simulink model "ECE552ProjectSim"  (R2018b)
settings: Solver=ode45  StartTime=0.0  StopTime=43200  RelTol=1e-3  EnableMultiTasking=on
undefined symbols (not defined in the file or in its folder): Acid, Lead, sigbuilder_block
libraries: powerlib x3, electricdrivelib x1, powerlib_meascontrol x1
settings Model: Creator=kegarcia  LastModifiedBy=cluck
settings SolverCC: ZeroCrossControl=DisableAll
settings DataIOCC: LimitDataPoints=on  SaveFormat=Array
settings OptimizationCC: LifeSpan=inf  SimCompilerOptimization=on
settings DebuggingCC: AlgebraicLoopMsg=none  MaxConsecutiveZCsMsg=none  SFUnexpectedBacktrackingDiag=warning  SFNoUnconditionalDefaultTransitionDiag=warning  SFExecutionAtInitializationDiag=none
settings HardwareCC: ProdBitPerPointer=32  ProdBitPerSizeT=32  ProdBitPerPtrDiffT=32  ProdLargestAtomicFloat=None  ProdIntDivRoundTo=Undefined  ProdEndianess=Unspecified  ProdWordSize=32  ProdHWDeviceType=32-bit Generic
settings ModelReferenceCC: PropagateSignalLabelsOutOfModel=off
settings SFSimCC: SimUseLocalCustomCode=off
settings RTWCC: RTWUseLocalCustomCode=off
settings CodeAppCC: StateflowObjectComments=on
settings GRTTargetCC: TargetLangStandard=C89/C90 (ANSI)  GeneratePreprocessorConditionals=Disable all
settings ConfigComp: CovMetricSettings=dw  CovHtmlReporting=on  CovSaveCumulativeToWorkspaceVar=on  CovSaveSingleToWorkspaceVar=on  CovExternalEMLEnable=off
settings SimscapeCC: SimscapeNormalizeSystem=off

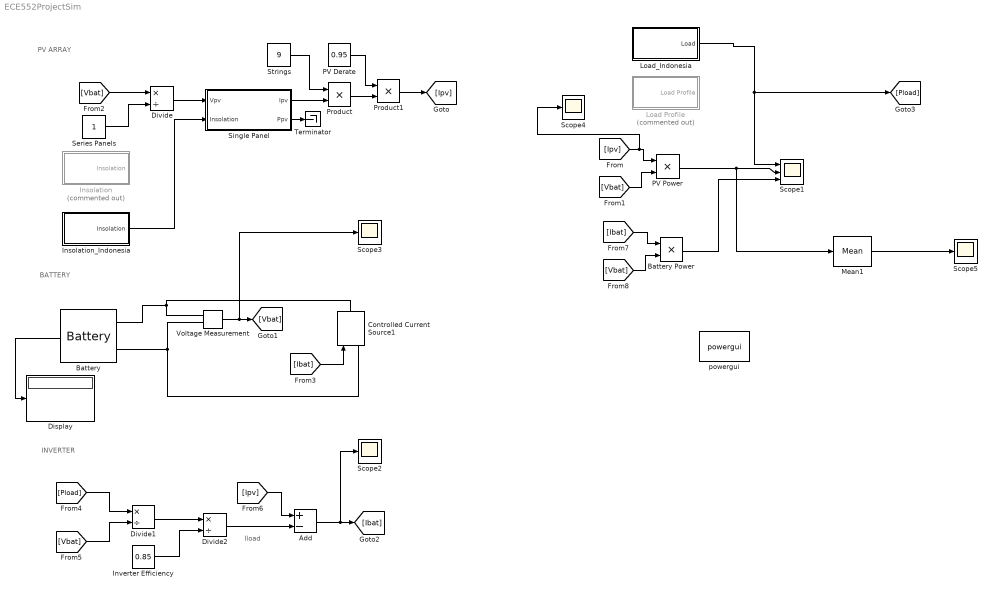
== system ECE552ProjectSim ==
  note: Iload
  note: INVERTER
  note: PV ARRAY
  note: BATTERY
  " Series Panels " : Constant
  " Strings" : Constant  Value=9
  Add : Sum  Inputs=+-
  Battery : electricdrivelib/Extra Sources/Battery  BatType=Lead-Acid  ShowTempParam=off  ThermalPreset=no  ShowAgeParam=off  NomV=24  NomQ=1200  SOC=95  Batt_Tr=30  PresetModel=off  MaxQ=1500  MinV=18  FullV=28  Dis_rate=5  R=0.0018462  Normal_OP=1200  expZone="[27        1500]"  current=[6.5 13 32.5]  Units=Time  Tci=20  NomT=20  T2=-30  MaxQ2=4.8  FullV2=7.1  Normal_OP2=5.655  expZone2="[6.58           1]"  Rca=0.6  ti=2000  Dp=0  Neq0=0  Tsim=1e6  Ta1=25  Qeol=5.4*0.9  Reol=0.013333*1.2  Char_age=[2.3478, 3]  Dis_age=[2.3478, 10]  N1=1500  N2=10500  N3=1000  N4=1400  Ta2=45  N5=950
      settings: SourceProductName=Simscape Electrical
  Battery Power : Product
  Controlled Current Source1 : powerlib/Electrical Sources/Controlled Current Source  Initialize=on  Source_Type=AC  Amplitude=0  Phase=0  Frequency=0  Measurements=None
      settings: SourceProductName=Simscape Electrical
  Display : Display
  Divide : Product  Inputs=*/
  Divide1 : Product  Inputs=*/
  Divide2 : Product  Inputs=*/
  Insolation : Subsystem  Tag=STV Subsys  Commented=on  LoadFcn=sigbuilder_block('load');  StartFcn=sigbuilder_block('start');  StopFcn=sigbuilder_block('stop');  ClipboardFcn=sigbuilder_block('clipboard');  mask(Sigbuilder block){tuvar=[0:10]}
      mask help: Simulink:masks:SigbuilderBlock_MD
      mask init:
      | if ~strcmp(get_param(bdroot(gcbh),'SimulationStatus'),'stopped') tuvar = sigbuilder_block('maskInit'); end
      settings: CopyFcn=sigbuilder_block('copy');  DeleteFcn=sigbuilder_block('delete');  ModelCloseFcn=sigbuilder_block('modelClose');  PreSaveFcn=sigbuilder_block('preSave');  PauseFcn=sigbuilder_block('pause')  ContinueFcn=sigbuilder_block('continue')  NameChangeFcn=sigbuilder_block('namechange');  OpenFcn=sigbuilder_block('open',[5.5 42.5 949 437.5 ]);  CloseFcn=sigbuilder_block('close');
      mask Display: plot(0, 0, 100, 100,[2, 2, 32, 32, 2], [68, 8, 8, 68, 68],[32, 2], [38, 38], [32, 19, 2],[53, 60, 44], [32, 17, 17, 2],[16, 16, 31, 31]);txt = getActiveGroup(gcbh);text(2, 100, txt,'verticalAlignment', 'top');
  Insolation_Indonesia : Subsystem  Tag=STV Subsys  LoadFcn=sigbuilder_block('load');  StartFcn=sigbuilder_block('start');  StopFcn=sigbuilder_block('stop');  ClipboardFcn=sigbuilder_block('clipboard');  mask(Sigbuilder block){tuvar=[0:10]}
      mask help: Simulink:masks:SigbuilderBlock_MD
      mask init:
      | if ~strcmp(get_param(bdroot(gcbh),'SimulationStatus'),'stopped') tuvar = sigbuilder_block('maskInit'); end
      settings: CopyFcn=sigbuilder_block('copy');  DeleteFcn=sigbuilder_block('delete');  ModelCloseFcn=sigbuilder_block('modelClose');  PreSaveFcn=sigbuilder_block('preSave');  PauseFcn=sigbuilder_block('pause');  ContinueFcn=sigbuilder_block('continue');  NameChangeFcn=sigbuilder_block('namechange');  OpenFcn=sigbuilder_block('open',[313.5 92 550.5 362.5 ]);  CloseFcn=sigbuilder_block('close');
      mask Display: plot(0, 0, 100, 100,[2, 2, 32, 32, 2], [68, 8, 8, 68, 68],[32, 2], [38, 38], [32, 19, 2],[53, 60, 44], [32, 17, 17, 2],[16, 16, 31, 31]);txt = getActiveGroup(gcbh);text(2, 100, txt,'verticalAlignment', 'top');
  Inverter Efficiency : Constant  Value=0.85
  Load Profile : Subsystem  Tag=STV Subsys  Commented=on  LoadFcn=sigbuilder_block('load');  StartFcn=sigbuilder_block('start');  StopFcn=sigbuilder_block('stop');  ClipboardFcn=sigbuilder_block('clipboard');  mask(Sigbuilder block){tuvar=[0:10]}
      mask help: Simulink:masks:SigbuilderBlock_MD
      mask init:
      | if ~strcmp(get_param(bdroot(gcbh),'SimulationStatus'),'stopped') tuvar = sigbuilder_block('maskInit'); end
      settings: CopyFcn=sigbuilder_block('copy');  DeleteFcn=sigbuilder_block('delete');  ModelCloseFcn=sigbuilder_block('modelClose');  PreSaveFcn=sigbuilder_block('preSave');  PauseFcn=sigbuilder_block('pause');  ContinueFcn=sigbuilder_block('continue');  NameChangeFcn=sigbuilder_block('namechange');  OpenFcn=sigbuilder_block('open',[97.5 52.5 543.5 351.5 ]);  CloseFcn=sigbuilder_block('close');
      mask Display: plot(0, 0, 100, 100,[2, 2, 32, 32, 2], [68, 8, 8, 68, 68],[32, 2], [38, 38], [32, 19, 2],[53, 60, 44], [32, 17, 17, 2],[16, 16, 31, 31]);txt = getActiveGroup(gcbh);text(2, 100, txt,'verticalAlignment', 'top');
  Load_Indonesia : Subsystem  Tag=STV Subsys  LoadFcn=sigbuilder_block('load');  StartFcn=sigbuilder_block('start');  StopFcn=sigbuilder_block('stop');  ClipboardFcn=sigbuilder_block('clipboard');  mask(Sigbuilder block){tuvar=[0:10]}
      mask help: Simulink:masks:SigbuilderBlock_MD
      mask init:
      | if ~strcmp(get_param(bdroot(gcbh),'SimulationStatus'),'stopped') tuvar = sigbuilder_block('maskInit'); end
      settings: CopyFcn=sigbuilder_block('copy');  DeleteFcn=sigbuilder_block('delete');  ModelCloseFcn=sigbuilder_block('modelClose');  PreSaveFcn=sigbuilder_block('preSave');  PauseFcn=sigbuilder_block('pause');  ContinueFcn=sigbuilder_block('continue');  NameChangeFcn=sigbuilder_block('namechange');  OpenFcn=sigbuilder_block('open',[313.5 92 550.5 362.5 ]);  CloseFcn=sigbuilder_block('close');
      mask Display: plot(0, 0, 100, 100,[2, 2, 32, 32, 2], [68, 8, 8, 68, 68],[32, 2], [38, 38], [32, 19, 2],[53, 60, 44], [32, 17, 17, 2],[16, 16, 31, 31]);txt = getActiveGroup(gcbh);text(2, 100, txt,'verticalAlignment', 'top');
  Mean1 : powerlib_meascontrol/Measurements/Mean  Freq=60  Vinit=0  Ts=0
      settings: SourceProductName=Simscape Electrical
  PV Derate : Constant  Value=0.95
  PV Power : Product
  Product : Product
  Product1 : Product
  Scope1 : Scope  NumInputPorts=3
  Scope2 : Scope
  Scope3 : Scope
  Scope4 : Scope
  Scope5 : Scope  NumInputPorts=3
  Single Panel : Subsystem  mask{Isc=9.71, Voc=39.5, Ir=9.07, Vr=31.2, Diode=on}
      mask prompts: Isc "Short-circuit current"; Voc "Open-circuit voltage"; Ir "Current at Pmax"; Vr "Voltage at Pmax"; Diode "By-pass diode?"
      mask help: PV module model based on module data-sheet parameters. This model has Vpv input, which is suitable for parallel connections of modules. Limitations: no temperature dependance, static model
      mask init:
      | % calculation of PV module parameters
      | % limitation: constant temperature
      | Ns = round(Voc/0.61); % default number of cells in series
      | Vt = 26e-3; % thermal voltage
      | G = Isc/1000; % irradiation to short-circuit current gain
      | Vmpc = Vr/Ns; % cell voltage at rated Pmax
      | Vocc = Voc/Ns; % cell open-circuit voltage
      | Rmpp = Vmpc/Ir; % cell load resistance at Pmax
      | %
      | Rp = 100*Vocc/Isc; % initial value for Rp
      | Vdm = Vocc; % initial value for Vdm
      | %
      | % iterative solution for model parameters: Io, Rs, Rp
      | for i=1:10
      | %
      |  Idm = Isc - Ir - Vdm/Rp; % pn-junction (diode) current at MPP
      |  Io = (Isc-Vocc/Rp)/(exp(Vocc/Vt)-1); % pn-junction reverse saturation current
      |  Vdm = Vt*log(Idm/Io+1); % pn-junction (diode) voltage at MPP
      |  Rs = (Vdm-Vmpc)/Ir; % cell series resistance
      |  Rd = (Rmpp - Rs)*Rp/(Rp-Rmpp+Rs); % diode incremental resistance at MPP
      |  Idm = Vt/Rd; % diode current at MPP based on incremental resistance
      |  Rp = Vdm/(Isc-Ir-Idm); % cell parallel resistance
      | %
      | end
      | %
      mask Display:
      | plot([0.3 0.4],[0.4 0.8]);
      | plot([0.4 0.5],[0.4 0.8]);
      | plot([0.5 0.6],[0.4 0.8]);
      | plot([0.6 0.7],[0.4 0.8]);
      | plot([0.3 0.6],[0.4 0.4]);
      | plot([0.325 0.625],[0.5 0.5]);
      | plot([0.35 0.65],[0.6 0.6]);
      | plot([0.375 0.675],[0.7 0.7]);
      | plot([0.4 0.7],[0.8 0.8]);
      | text(0.5,0.9,'PV module (V)','horizontalAlignment', 'center');
  Terminator : Terminator
  Voltage Measurement : powerlib/Measurements/Voltage Measurement  PhasorSimulation=off  OutputType=Complex  PSBequivalent=0
      settings: SourceProductName=Simscape Electrical
  powergui : powerlib/powergui  Priority=1  SimulationMode=Discrete  SampleTime=10  frequency=60  Iterations=50  frequencyindice=0  Pbase=100e6  ErrMax=1e-4  UnitsV=kV  UnitsW=MW  buscounter=0  FunctionMessages=off  echomessages=off  EnableUseOfTLC=off  CurrentSourceSwitches=off  DisableSnubberDevices=off  DisableRonSwitches=off  DisableVfSwitches=off  DisplayEquations=off  SolverType=Tustin  Interpol=off  ExternalGateDelay=off  methode=off  Ts=0  x0status=blocks  SPID=off  SwTol=0  HookPort=off  RestoreLinks=warning  ResistiveCurrentMeasurement=off  Frange=[0:2:500]  Ylog=off  Xlog=on  ShowGrid=off  save=off  variable=ZData  structure=0  ZoomFFT=off  StartTime=0.0  cycles=1  DisplayStyle=1  fundamental=60  FreqAxis=off  MaxFrequency=1000  frequencyindicesteady=1  RmsSteady=1  display=off
  wires:
  Divide/1 -> Single Panel/1(Vpv)
  " Series Panels "/1 -> Divide/2
  " Strings"/1 -> Product/1
  Single Panel/1(Ipv) -> Product/2
  Product/1 -> Product1/2
  PV Derate/1 -> Product1/1
  Product1/1 -> [Ipv]
  [Ipv] -> Scope4/1, PV Power/1
  PV Power/1 -> Mean1/1, Scope1/2
  [Vbat] -> PV Power/2
  Voltage Measurement/1 -> Scope3/1, [Vbat]
  [Vbat] -> Divide/1
  Single Panel/2(Ppv) -> Terminator/1
  [Ibat] -> Controlled Current Source1/1
  [Pload] -> Divide1/1
  [Vbat] -> Divide1/2
  Divide1/1 -> Divide2/1
  Divide2/1 -> Add/2
  [Ipv] -> Add/1
  Add/1 -> Scope2/1, [Ibat]
  [Ibat] -> Battery Power/1
  [Vbat] -> Battery Power/2
  Battery Power/1 -> Scope1/3
  Insolation_Indonesia/1(Insolation) -> Single Panel/2(Insolation)
  Load_Indonesia/1(Load) -> Scope1/1, [Pload]
  Battery/1 -> Display/1
  Inverter Efficiency/1 -> Divide2/2
  Mean1/1 -> Scope5/2
  connections:
  Voltage Measurement/LConn1 -- Battery/LConn1 -- Controlled Current Source1/RConn1
  Voltage Measurement/LConn2 -- Controlled Current Source1/LConn1 -- Battery/LConn2

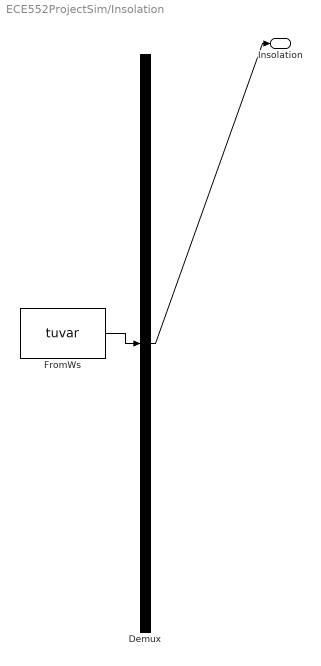
== system ECE552ProjectSim/Insolation ==
  Demux : Demux  Tag=STV Demux  Outputs=1
  FromWs : FromWorkspace  Tag=STV FromWs  VariableName=tuvar  SampleTime=0
      SigBuilderData=|
      | common.afterFinalStr = 'Extrapolate'
      | common.sampleTime = 0
      | dataSet.timeRange = [0 46800]
      | dataSet.name = 'Imported_Group 1'
      | sbobj.Name = 'Signal Builder'
      | sbobj.Groups.Name = 'Imported_Group 1'
      | sbobj.Groups.Signals.Name = 'Insolation'
      | sbobj.Groups.Signals.XData = [0 3600 3600 7200 7200 10800 10800 14400 14400 18000 18000 21600 21600 25200 25200 28800 28800 32400 32400 36000 36000 39600 39600 43200 43200 46800]
      | sbobj.Groups.Signals.YData = [0 0 34.8 34.8 158.2 158.2 199.82 199.82 241.92 241.92 766.21 766.21 722.78 722.78 566.04 566.04 607.59 607.559 231.99 231.99 79.08 79.08 7.9 7.9 0 0]
      | sbobj.Groups.TimeRange = [0 46800]
  Insolation : Outport
  wires:
  Demux/1 -> Insolation/1
  FromWs/1 -> Demux/1

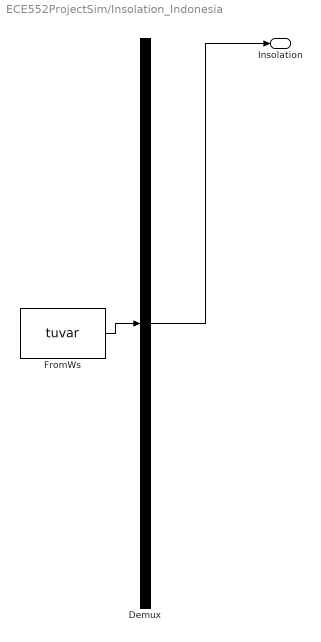
== system ECE552ProjectSim/Insolation_Indonesia ==
  Demux : Demux  Tag=STV Demux  Outputs=1
  FromWs : FromWorkspace  Tag=STV FromWs  VariableName=tuvar  SampleTime=0
      SigBuilderData=|
      | common.afterFinalStr = 'Extrapolate'
      | common.sampleTime = 0
      | dataSet.timeRange = [0 604200]
      | dataSet.name = 'Imported_Group 1'
      | sbobj.Groups.Name = 'Imported_Group 1'
      | sbobj.Groups.Signals.Name = 'Insolation'
      | sbobj.Groups.Signals.XData = [0 600 1200 1800 2400 3000 3600 4200 4800 5400 6000 6600 ... (1008 elements, 1x1008)]
      | sbobj.Groups.Signals.YData = [0 0 0 0 0 0 0 0 0 0 0 0 ... (1008 elements, 1x1008)]
      | sbobj.Groups.TimeRange = [0 604200]
  Insolation : Outport  Tag=STV Outport
  wires:
  Demux/1 -> Insolation/1
  FromWs/1 -> Demux/1

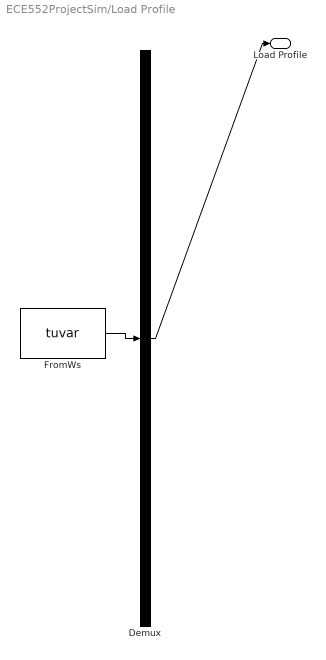
== system ECE552ProjectSim/Load Profile ==
  Demux : Demux  Tag=STV Demux  Outputs=1
  FromWs : FromWorkspace  Tag=STV FromWs  VariableName=tuvar  SampleTime=0
      SigBuilderData=|
      | common.afterFinalStr = 'Extrapolate'
      | common.sampleTime = 0
      | dataSet.timeRange = [0 43200]
      | dataSet.name = 'Imported_Group 1'
      | sbobj.Name = 'Signal Builder'
      | sbobj.Groups.Name = 'Imported_Group 1'
      | sbobj.Groups.Signals.Name = 'Load Profile'
      | sbobj.Groups.Signals.XData = [0 3600 3600 7200 7200 10800 10800 14400 14400 18000 18000 21600 21600 25200 25200 28800 32400 32400 36000 39600 43200]
      | sbobj.Groups.Signals.YData = [0 0 101.9 101.9 160.7 160.7 351.4 351.4 225.4 225.4 201.8 201.8 101.8 101.8 125.4 125.4 125.4 101.8 101.8 101.8 101.8]
      | sbobj.Groups.TimeRange = [0 43200]
  Load Profile : Outport
  wires:
  FromWs/1 -> Demux/1
  Demux/1 -> Load Profile/1

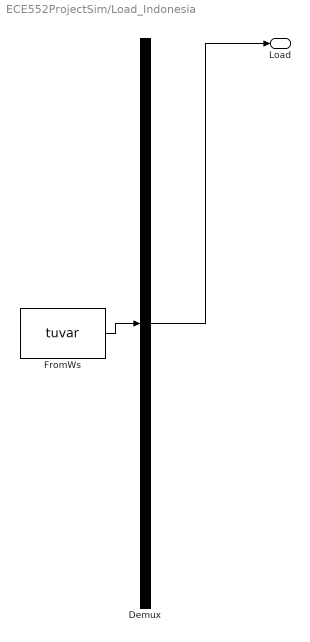
== system ECE552ProjectSim/Load_Indonesia ==
  Demux : Demux  Tag=STV Demux  Outputs=1
  FromWs : FromWorkspace  Tag=STV FromWs  VariableName=tuvar  SampleTime=0
      SigBuilderData=|
      | common.afterFinalStr = 'Extrapolate'
      | common.sampleTime = 0
      | dataSet.timeRange = [0 604200]
      | dataSet.name = 'Imported_Group 1'
      | sbobj.Groups.Name = 'Imported_Group 1'
      | sbobj.Groups.Signals.Name = 'Load'
      | sbobj.Groups.Signals.XData = [0 600 1200 1800 2400 3000 3600 4200 4800 5400 6000 6600 ... (1036 elements, 1x1036)]
      | sbobj.Groups.Signals.YData = [6.34936 6.34936 6.34936 6.34936 6.34936 6.34936 6.34936 6.34936 6.34936 6.34936 6.34936 6.34936 ... (1036 elements, 1x1036)]
      | sbobj.Groups.TimeRange = [0 604200]
  Load : Outport  Tag=STV Outport
  wires:
  Demux/1 -> Load/1
  FromWs/1 -> Demux/1

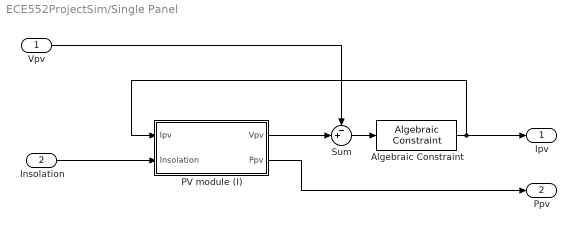
== system ECE552ProjectSim/Single Panel ==
  Vpv : Inport
  Insolation : Inport  Port=2
  Algebraic Constraint : AlgebraicConstraint  InitialGuess=5
  PV module (I) : Subsystem
  Sum : Sum  Inputs=-+|
  Ipv : Outport
  Ppv : Outport  Port=2
  wires:
  Insolation/1 -> PV module (I)/2(Insolation)
  PV module (I)/1(Vpv) -> Sum/2
  Sum/1 -> Algebraic Constraint/1
  Algebraic Constraint/1 -> Ipv/1, PV module (I)/1(Ipv)
  Vpv/1 -> Sum/1
  PV module (I)/2(Ppv) -> Ppv/1

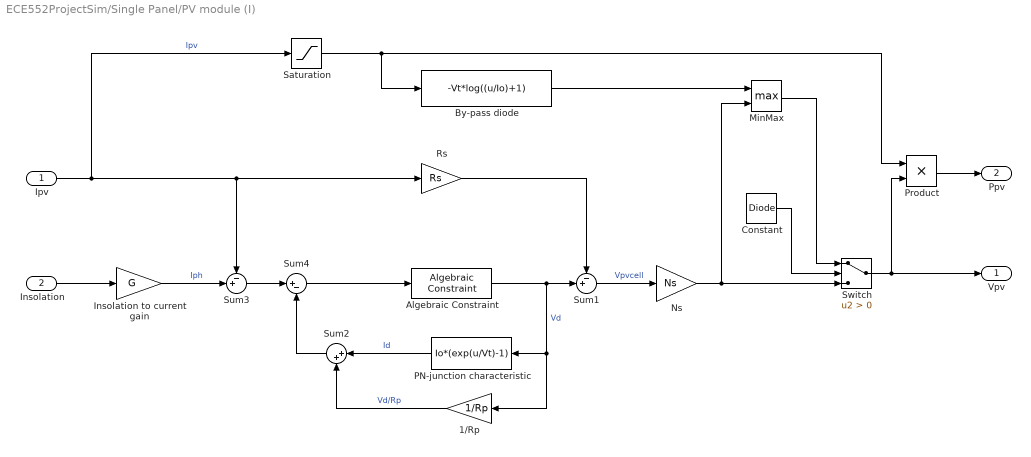
== system ECE552ProjectSim/Single Panel/PV module (I) ==
  Ipv : Inport
  Insolation : Inport  Port=2
  1/Rp : Gain  Gain=1/Rp
  Algebraic Constraint : AlgebraicConstraint  InitialGuess=0.1
  By-pass diode : Fcn  Expr=-Vt*log((u/Io)+1)
  Constant : Constant  Value=Diode
  Insolation to current gain : Gain  Gain=G
  MinMax : MinMax  Function=max  Inputs=2
  Ns : Gain  Gain=Ns
  PN-junction characteristic : Fcn  Expr=Io*(exp(u/Vt)-1)
  Product : Product  RndMeth=Zero
  Rs : Gain  Gain=Rs
  Saturation : Saturate  UpperLimit=inf  LowerLimit=0
  Sum1 : Sum  Inputs=-+|
  Sum2 : Sum  Inputs=|++
  Sum3 : Sum  Inputs=-+|
  Sum4 : Sum  Inputs=|+-
  Switch : Switch  Criteria=u2 > Threshold
  Vpv : Outport
  Ppv : Outport  Port=2
  wires:
  Insolation/1 -> Insolation to current gain/1
  Insolation to current gain/1 -> Sum3/2  "Iph"
  Ipv/1 -> Saturation/1, Sum3/1, Rs/1  "Ipv"
  Product/1 -> Ppv/1
  Sum4/1 -> Algebraic Constraint/1
  Algebraic Constraint/1 -> Sum1/2, 1/Rp/1, PN-junction characteristic/1  "Vd"
  Sum1/1 -> Ns/1  "Vpvcell"
  Rs/1 -> Sum1/1
  By-pass diode/1 -> MinMax/1
  Ns/1 -> MinMax/2, Switch/3
  MinMax/1 -> Switch/1
  Constant/1 -> Switch/2
  Switch/1 -> Vpv/1, Product/2
  Saturation/1 -> Product/1, By-pass diode/1
  Sum3/1 -> Sum4/1
  Sum2/1 -> Sum4/2
  PN-junction characteristic/1 -> Sum2/1  "Id"
  1/Rp/1 -> Sum2/2  "Vd/Rp"
